simulink model "SimulationTest"  (R2016a)
settings: Solver=FixedStepDiscrete  StartTime=0.0  StopTime=500  FixedStep=sCoreParams.core.stepPeriod  RelTol=1e-3
values from neighbouring files (symbols this model uses):
  sCoreParams = InitCoreParams_Dependent(sCoreParams)    [initializationScript.m]
libraries: dspsrcs4 x2, simulink x1
settings Model: Creator=rzelmann  LastModifiedBy=rzelmann
settings OptimizationCC: DefaultParameterBehavior=Inlined  InlineInvariantSignals=on

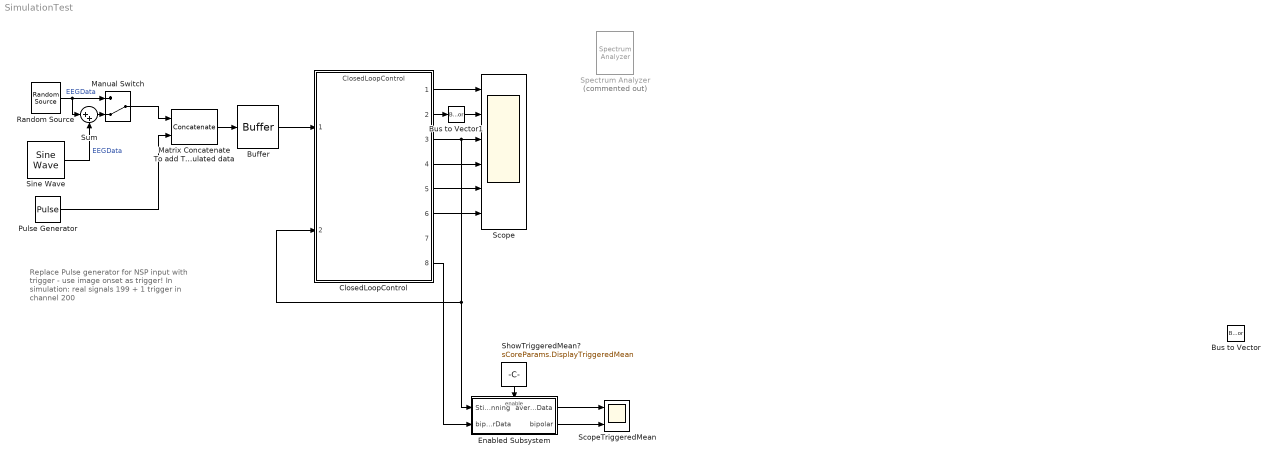
== system SimulationTest ==
  note: Replace Pulse generator for NSP
      | input with trigger - use image onset as trigger!
      | In simulation: real signals 199 + 1 trigger in channel 200
  Buffer : Buffer  N=2  V=1  TreatMby1Signals=One channel  OutputFrames=off
  Bus to Vector : BusToVector
  Bus to Vector1 : BusToVector
  ClosedLoopControl : ModelReference  ModelNameDialog=ClosedLoopControl  SimulationMode=Normal  ModelReferenceVersion=1.102
  Enabled Subsystem : Subsystem  TreatAsAtomicUnit=on
  Manual Switch : ManualSwitch  CurrentSetting=0
  Matrix Concatenate To add Trigger after simulated data : Concatenate  Mode=Multidimensional array  ConcatenateDimension=2
  Pulse Generator : DiscretePulseGenerator  Period=sCoreParams.core.samplingRate * 10  SampleTime=sCoreParams.core.stepPeriod  VectorParams1D=off
  Random Source : dspsrcs4/Random Source  SrcType=Uniform  NormMethod=Ziggurat  CltLength=12  MinVal=-10 * ones(1, sCoreParams.core.maxChannelsPerNSP-1)  MaxVal=10 * ones(1, sCoreParams.core.maxChannelsPerNSP-1)  MeanVal=0  VarVal=1  RepMode=Not repeatable  rawSeed=1  IsInherit=off  SampMode=Discrete  SampTime=sCoreParams.core.stepPeriod  SampFrame=1  DataType=Double  OutComplex=Real  OutputFrames=off
  Scope : Scope  NumInputPorts=6
  ScopeTriggeredMean : Scope  NumInputPorts=2
  ShowTriggeredMean? : Constant  Value=sCoreParams.DisplayTriggeredMean
  Sine Wave : dspsrcs4/Sine Wave  Amplitude=100 * ones(1, sCoreParams.core.maxChannelsPerNSP-1)  Frequency=80  Phase=rand(1, sCoreParams.core.maxChannelsPerNSP-1)  SampleMode=Discrete  OutComplex=Real  CompMethod=Trigonometric fcn  TableSize=Speed  SampleTime=sCoreParams.core.stepPeriod  SamplesPerFrame=1  ResetState=Restart at time zero  OutputFrames=off  dataType=double  wordLen=16  udDataType=sfix(16)  fracBitsMode=Best precision  numFracBits=15  OutDataTypeStr=double  LastOutDataTypeStr=double
  Spectrum Analyzer : SpectrumAnalyzer  Commented=on
  Sum : Sum  Inputs=|++
  wires:
  Random Source/1 -> Sum/1, Manual Switch/1  "EEGData"
  ClosedLoopControl/1 -> Scope/1
  ClosedLoopControl/2 -> Bus to Vector1/1
  ClosedLoopControl/3 -> ClosedLoopControl/2, Enabled Subsystem/1(StimHappenning), Scope/3
  ClosedLoopControl/4 -> Scope/4
  ClosedLoopControl/5 -> Scope/5
  ClosedLoopControl/6 -> Scope/6
  Buffer/1 -> ClosedLoopControl/1
  Manual Switch/1 -> Matrix Concatenate To add Trigger after simulated data/1
  Pulse Generator/1 -> Matrix Concatenate To add Trigger after simulated data/2
  Matrix Concatenate To add Trigger after simulated data/1 -> Buffer/1
  Enabled Subsystem/1(averagedData) -> ScopeTriggeredMean/1
  ClosedLoopControl/8 -> Enabled Subsystem/2(bipolarData)
  ShowTriggeredMean?/1 -> Enabled Subsystem/Enable
  Sine Wave/1 -> Sum/2  "EEGData"
  Enabled Subsystem/2(bipolar) -> ScopeTriggeredMean/2
  Sum/1 -> Manual Switch/2
  Bus to Vector1/1 -> Scope/2

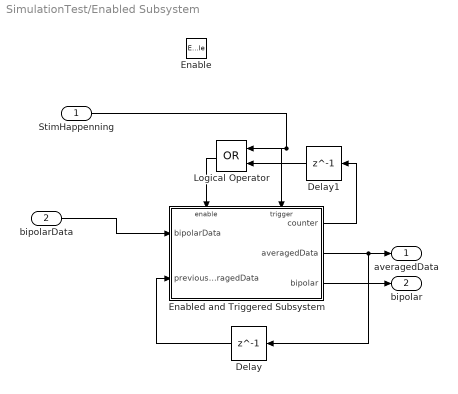
== system SimulationTest/Enabled Subsystem ==
  StimHappenning : Inport  OutDataTypeStr=boolean
  bipolarData : Inport  Port=2
  Enable : EnablePort
  Delay : Delay  DelayLength=1
  Delay1 : Delay  DelayLength=1
  Enabled and Triggered Subsystem : Subsystem  TreatAsAtomicUnit=on
  Logical Operator : Logic  Operator=OR  AllPortsSameDT=off  OutDataTypeStr=boolean
  averagedData : Outport
  bipolar : Outport  Port=2
  wires:
  Delay/1 -> Enabled and Triggered Subsystem/2(previousAveragedData)
  bipolarData/1 -> Enabled and Triggered Subsystem/1(bipolarData)
  Enabled and Triggered Subsystem/2(averagedData) -> Delay/1, averagedData/1
  StimHappenning/1 -> Logical Operator/1, Enabled and Triggered Subsystem/Trigger
  Logical Operator/1 -> Enabled and Triggered Subsystem/Enable
  Enabled and Triggered Subsystem/1(counter) -> Delay1/1
  Delay1/1 -> Logical Operator/2
  Enabled and Triggered Subsystem/3(bipolar) -> bipolar/1

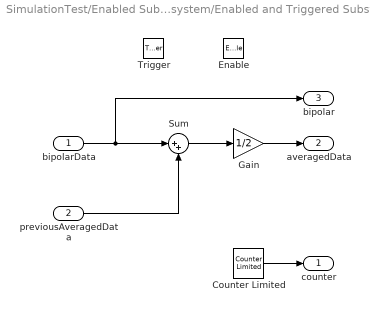
== system SimulationTest/Enabled Subsystem/Enabled and Triggered Subsystem ==
  bipolarData : Inport
  previousAveragedData : Inport  Port=2
  Enable : EnablePort
  Trigger : TriggerPort  VariantControl=Variant
  Counter Limited : simulink/Sources/Counter Limited  uplimit=sCoreParams.DurationTriggeredMeanFrames  tsamp=-1
  Gain : Gain  Gain=1/2
  Sum : Sum  Inputs=|++
  counter : Outport
  averagedData : Outport  Port=2  InitialOutput=zeros(sCoreParams.FrameSize,sCoreParams.decoders.txDetector.nChannels)
  bipolar : Outport  Port=3
  wires:
  bipolarData/1 -> bipolar/1, Sum/1
  Sum/1 -> Gain/1
  previousAveragedData/1 -> Sum/2
  Gain/1 -> averagedData/1
  Counter Limited/1 -> counter/1
